simulink model "A2_4_PID_angle_with_saturation"  (Simulink 7.4)
settings: Solver=FixedStepDiscrete  StartTime=0.0  StopTime=10  RelTol=1e-3
undefined symbols (not defined in the file): dend, gamma, Kp, numd, Td, Ti
libraries: DCmotor_library x1
settings Model: Creator=Natalia  LastModifiedBy=ma
settings DebuggingCC: StrictBusMsg=ErrorLevel1
settings HardwareCC: ProdIntDivRoundTo=Zero  ProdEndianess=LittleEndian  ProdHWDeviceType=Generic->32-bit x86 compatible
settings RTWCC: SystemTargetFile=rtwin.tlc  TemplateMakefile=rtwin.tmf  Description=Real-Time Windows Target  ProcessScript=rtwin_make_rtw_hook  RTWCompilerOptimization=On
settings CodeAppCC: MaxIdLength=95  CustomSymbolStrType=$N$R$M_T
settings TargetCC: TargetLibSuffix=_rtwin.lib  TargetPreCompLibLocation=C:\Program Files\MATLAB\R2012b\toolbox\rtw\targets\rtwin\lib\win64  TargetFunctionLibrary=ANSI_C  IsPILTarget=off  MatFileLogging=on  EnableShiftOperators=on
settings CustomProperty: DataType=string  Value=C:/PROGRA~1/MATLAB/R2012b/toolbox/rtw/targets/rtwin

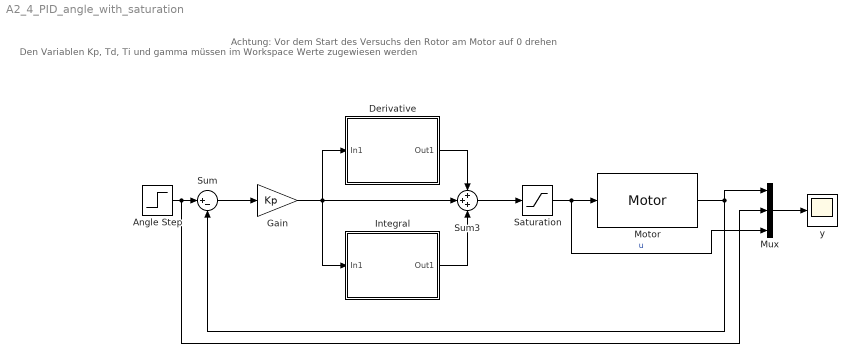
== system A2_4_PID_angle_with_saturation ==
  note: Den Variablen
      | Kp, Td, Ti und gamma
      | müssen im Workspace
      | Werte zugewiesen werden
  note: Achtung:
      | Vor dem Start des Versuchs
      | den Rotor am Motor auf 0 drehen
  Angle Step : Step  After=2*pi  SampleTime=0.01
  Derivative : Subsystem  mask(DiscretizedTransferFcn){Numerator=[Td 0], Denominator=[gamma*Td 1], AbsTol=auto, SampleTime=0.01, method=tustin, Wc=1}
      mask prompts: Numerator "Numerator (enter in s-domain:)"; Denominator "Denominator (enter in s-domain:)"; AbsTol "Absolute tolerance:"; SampleTime "Sample time:"; Wc "Critical Frequency (Hz):"
      mask help: Continuous mask uses c2d to transform parameters onto the Discrete Transfer function block inside.
      mask init:
      | st=SampleTime;
      | if length(st)>1
      |     st=SampleTime(1);
      | end
      | if(st>0)
      |     [numd,dend] = sldiscutil('disctransferfcn',{st,method,Wc,Numerator,Denominator});
      | end	
      | s = get_param(gcb,'maskvalues');
      | nums = s{1};
      | dens = s{2};
      | %numc = eval(nums);
      | %denc = eval(dens);
      | sldiscutil('inittfmask', st);
      | if(st==0)
      | set_param([gcb '/Transfer Fcn'], 'AbsoluteTolerance', AbsTol);
      | end
      mask StyleString: edit,edit,edit,edit,popup(zoh|foh|tustin|prewarp|matched),edit
      mask CallbackString: ||||hidecrit|
      mask Display:
      | dpoly(nums,dens)
      | text( 0.5, 1.0, method, 'verticalAlignment','top')
  Gain : Gain  Gain=Kp
  Integral : Subsystem  mask(DiscretizedTransferFcn){Numerator=[1], Denominator=[Ti 0], AbsTol=auto, SampleTime=0.01, method=tustin, Wc=1}
      mask prompts: Numerator "Numerator (enter in s-domain:)"; Denominator "Denominator (enter in s-domain:)"; AbsTol "Absolute tolerance:"; SampleTime "Sample time:"; Wc "Critical Frequency (Hz):"
      mask help: Continuous mask uses c2d to transform parameters onto the Discrete Transfer function block inside.
      mask init: same as A2_4_PID_angle_with_saturation/Derivative
      mask StyleString: edit,edit,edit,edit,popup(zoh|foh|tustin|prewarp|matched),edit
      mask CallbackString: ||||hidecrit|
      mask Display:
      | dpoly(nums,dens)
      | text( 0.5, 1.0, method, 'verticalAlignment','top')
  Motor : DCmotor_library/Motor  motoridinput=1  name_signal=Angle  ts=10
  Mux : Mux  Inputs=3
  Saturation : Saturate  UpperLimit=7  LowerLimit=-7
  Sum : Sum  Inputs=|+-
  Sum3 : Sum  Inputs=+++
  y : Scope
      settings: YMin=-3  YMax=13
  wires:
  Angle Step/1 -> Mux/2, Sum/1
  Gain/1 -> Derivative/1(In1), Sum3/2, Integral/1(In1)
  Sum/1 -> Gain/1
  Derivative/1(Out1) -> Sum3/1
  Motor/1 -> Mux/1, Sum/2
  Integral/1(Out1) -> Sum3/3
  Mux/1 -> y/1
  Sum3/1 -> Saturation/1
  Saturation/1 -> Mux/3, Motor/1  "u"

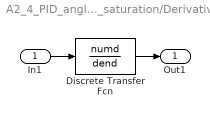
== system A2_4_PID_angle_with_saturation/Derivative ==
  In1 : Inport
  Discrete Transfer Fcn : DiscreteTransferFcn  Numerator=numd  Denominator=dend  SampleTime=SampleTime
  Out1 : Outport
  wires:
  In1/1 -> Discrete Transfer Fcn/1
  Discrete Transfer Fcn/1 -> Out1/1

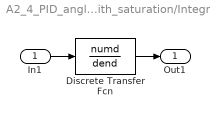
== system A2_4_PID_angle_with_saturation/Integral ==
  In1 : Inport
  Discrete Transfer Fcn : DiscreteTransferFcn  Numerator=numd  Denominator=dend  SampleTime=SampleTime
  Out1 : Outport
  wires:
  Discrete Transfer Fcn/1 -> Out1/1
  In1/1 -> Discrete Transfer Fcn/1
